simulink model "MultiObj_LTI_01_sim"  (R2018b)
settings: Solver=FixedStepAuto  StartTime=0.0  StopTime=10.0  FixedStep=0.01  MaxStep=0.01  RelTol=1e-3  EnableMultiTasking=on
values from neighbouring files (symbols this model uses):
  A = 1/sqrt(h)    [MultiObj_LTI_01.m]    (also in MultiObj_LTI_02.m = [0        0       1        0;      0        0       0       )
  G = ss(A,B,C,D)    [MultiObj_LTI_01.m]    (also in MultiObj_LTI_02.m)
  h = 0.01    [MultiObj_LTI_01.m]
libraries: cstblocks x2
settings Model: Creator=ferna  LastModifiedBy=ferna
settings OptimizationCC: LifeSpan=inf
settings DebuggingCC: SFUnexpectedBacktrackingDiag=warning  SFNoUnconditionalDefaultTransitionDiag=warning
settings SFSimCC: SimUseLocalCustomCode=off
settings RTWCC: RTWUseLocalCustomCode=off
settings CodeAppCC: StateflowObjectComments=on
settings GRTTargetCC: TargetLangStandard=C89/C90 (ANSI)  GeneratePreprocessorConditionals=Disable all
settings ConfigComp: CovMetricSettings=dw  CovHtmlReporting=on  CovSaveCumulativeToWorkspaceVar=on  CovSaveSingleToWorkspaceVar=on  CovExternalEMLEnable=off

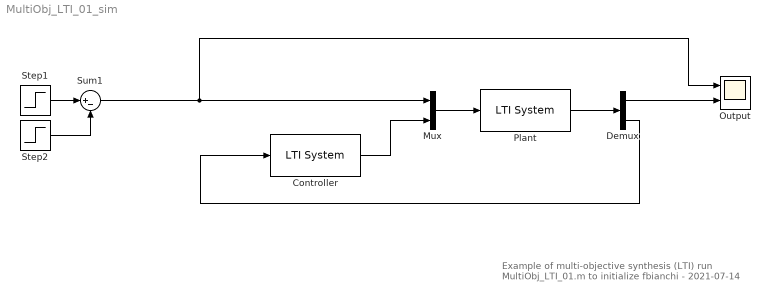
== system MultiObj_LTI_01_sim ==
  note: Example of multi-objective synthesis (LTI)
      | run MultiObj_LTI_01.m to initialize
      |
      | fbianchi - 2021-07-14
  Controller : cstblocks/LTI System  sys=Klpv_h2g  IC=[]
  Demux : Demux  Outputs=[3 1]
  Mux : Mux  Inputs=2
  Output : Scope  NumInputPorts=2
  Plant : cstblocks/LTI System  sys=G(3:6,:)  IC=[]
  Step1 : Step  Time=0  After=A  SampleTime=0
  Step2 : Step  Time=h  After=A  SampleTime=0
  Sum1 : Sum  Inputs=|+-
  wires:
  Step1/1 -> Sum1/1
  Step2/1 -> Sum1/2
  Sum1/1 -> Output/1, Mux/1
  Mux/1 -> Plant/1
  Controller/1 -> Mux/2
  Plant/1 -> Demux/1
  Demux/2 -> Controller/1
  Demux/1 -> Output/2
